simulink model "temp_model_1"  (R2023b)
settings: Solver=FixedStepDiscrete  StartTime=0.0  StopTime=10.0  RelTol=1e-3
values from neighbouring files (symbols this model uses):
  T_a_1 = 0.9832    [iterate_gains.m]
  T_b_1 = 0.03446    [iterate_gains.m]
settings Model: Creator=john  LastModifiedBy=john

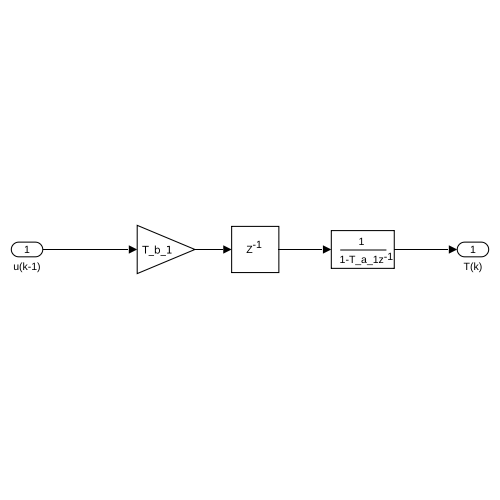
[thumbnail: Simulink's stored preview of the top-level diagram]
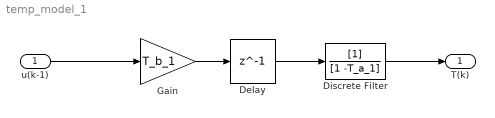
== system temp_model_1 ==
  u(k-1) : Inport
  Delay : Delay  DelayLength=1  SampleTime=1
  Discrete Filter : DiscreteFilter  Denominator=[1 -T_a_1]
  Gain : Gain  Gain=T_b_1
  T(k) : Outport
  wires:
  Delay/1 -> Discrete Filter/1
  u(k-1)/1 -> Gain/1
  Discrete Filter/1 -> T(k)/1
  Gain/1 -> Delay/1
